simulink model "Epm"  (Simulink 8.4)
settings: Solver=ode45  StartTime=0.0  StopTime=10.0  RelTol=1e-3
settings Model: Creator=ric9fe  LastModifiedBy=ric9fe
settings OptimizationCC: ExpressionDepthLimit=128
settings DebuggingCC: UnderspecifiedInitializationDetection=Simplified  MergeDetectMultiDrivingBlocksExec=error  FcnCallInpInsideContextMsg=EnableAllAsWarning  StateNameClashWarn=none

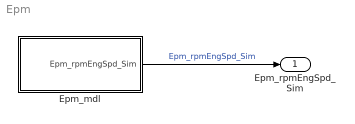
== system Epm ==
  Epm_mdl : Subsystem
  Epm_rpmEngSpd_Sim : Outport
  wires:
  Epm_mdl/1(Epm_rpmEngSpd_Sim) -> Epm_rpmEngSpd_Sim/1  "Epm_rpmEngSpd_Sim"

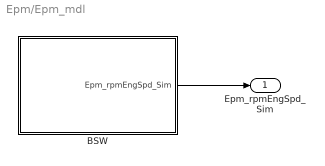
== system Epm/Epm_mdl ==
  BSW : Subsystem
  Epm_rpmEngSpd_Sim : Outport
  wires:
  BSW/1(Epm_rpmEngSpd_Sim) -> Epm_rpmEngSpd_Sim/1

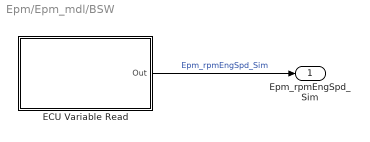
== system Epm/Epm_mdl/BSW ==
  ECU Variable Read : Subsystem  Tag=ECU_MsmtVariable_Read  Description=|  AncestorBlock=ehooks_lib/Library Blocks/ECU Variable Read  mask(ECU_MsmtVariable_Read){PortName=Epm_nEngCurr, DataTypeName=double, VariableName=Epm_nEngCurr, DisplayName=Epm_nEngCurr, ElementIndex=-1, PerformConversion=on, UseDisplayName=off, AllowStorageReuse=off}
      | [$SL_INT_DD 20030]
      | EHOOKS ECU measurement variable single read block.
      mask prompts: PortName "Port name (name of the variable read)"; DataTypeName "Data type name (alias of the A2L data type)"; VariableName "Variable name (name of the measurement)"; DisplayName "Display name (display identifier of the measurement)"; ElementIndex "Element index (array variable index)"; PerformConversion "Perform value conversion (conversion flag)"; UseDisplayName "Use display name (display name usage flag)"; AllowStorageReuse "Allow port storage reuse (enable data merge block support)"
      mask help:
      | EHOOKS ECU measurement variable single read block (ECU single read block).
      |
      | The ECU single read block allows Simulink models to read from an existing ECU variable. Note that the block parameters can only be changed via the EHOOKS configuration GUI and the specialized EHOOKS automation API functions.
      settings: AttributesFormatString=Variable: 'Epm_nEngCurr'
      mask Display: port_label('Output', 1, 'Epm_nEngCurr (phys)')
  Epm_rpmEngSpd_Sim : Outport
  wires:
  ECU Variable Read/1(Out) -> Epm_rpmEngSpd_Sim/1  "Epm_rpmEngSpd_Sim"

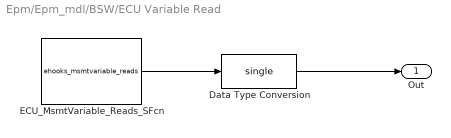
== system Epm/Epm_mdl/BSW/ECU Variable Read ==
  Data Type Conversion : DataTypeConversion  OutDataTypeStr=single  RndMeth=Nearest
  ECU_MsmtVariable_Reads_SFcn : S-Function  Tag=ECU_MsmtVariable_Reads_SFcn  Description=Internal S-function for custom block ECU_MsmtVariable_Reads and custom block ECU_BackupMsmtVariable_Reads. Do not rename!  FunctionName=ehooks_msmtvariable_reads  Parameters=uint8(NoOutputPorts), OutputPortDataTypes, PortStorageReuse, VariableNames, ElementIndexes, ConversionModes  EnableBusSupport=off  mask(ECU_MsmtVariable_Reads_SFcn){NoOutputPorts=1, PortStorageReuse=0, OutputPortNames=Epm_nEngCurr, OutputPortDataTypes=double, VariableNames=Epm_nEngCurr, ElementIndexes=-1, ConversionModes=phys}
      mask prompts: NoOutputPorts "Number of output ports"; PortStorageReuse "Enable port storage reuse"; OutputPortNames "Output port names"; OutputPortDataTypes "Output port data types"; VariableNames "Variable C names"; ElementIndexes "Variable element indexes"; ConversionModes "Conversion modes"
      mask help: Internal S-function for custom block ECU_MsmtVariable_Reads and custom block ECU_BackupMsmtVariable_Reads. Do not rename!
      mask Display: disp('EHOOKS ECU\nVariable Reads\nS-Function')
  Out : Outport
  wires:
  ECU_MsmtVariable_Reads_SFcn/1 -> Data Type Conversion/1
  Data Type Conversion/1 -> Out/1
